simulink model "EncoderTrackingLoop"  (R2022a)
settings: Solver=ode4  StartTime=0.0  StopTime=inf  FixedStep=1/100  RelTol=1e-3
undefined symbols (not defined in the file): DiscIntNeverNeededParam, National_Instruments, PCI
libraries: sldrtlib x3, simulink x2
settings Model: Creator=UTFPR  LastModifiedBy=ederh
settings DebuggingCC: UnconnectedInputMsg=warning  UnconnectedOutputMsg=warning  UnconnectedLineMsg=warning
settings HardwareCC: ProdBitPerLong=64  ProdHWDeviceType=Intel->x86-64 (Linux 64)
settings RTWCC: Description=Simulink Desktop Real-Time  SystemTargetFile=sldrt.tlc  TemplateMakefile=sldrt.tmf  RTWCompilerOptimization=on  DLArmComputeVersion=19.05
settings CodeAppCC: MaxIdLength=95
settings SimulinkDesktopRealTimeCC: TargetLibSuffix=_sldrt.a  TargetPreCompLibLocation=C:\Program Files\MATLAB\R2022a\toolbox\sldrt\lib\win64

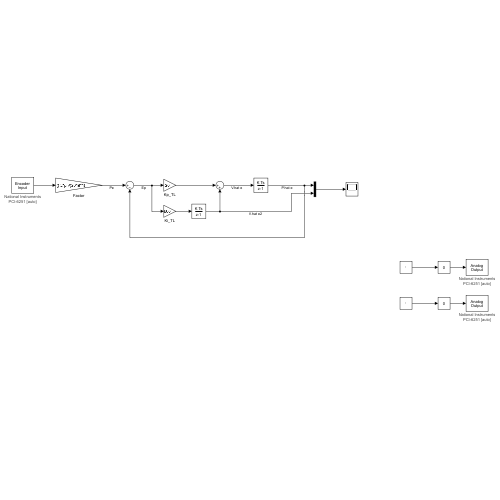
[thumbnail: Simulink's stored preview of the top-level diagram]
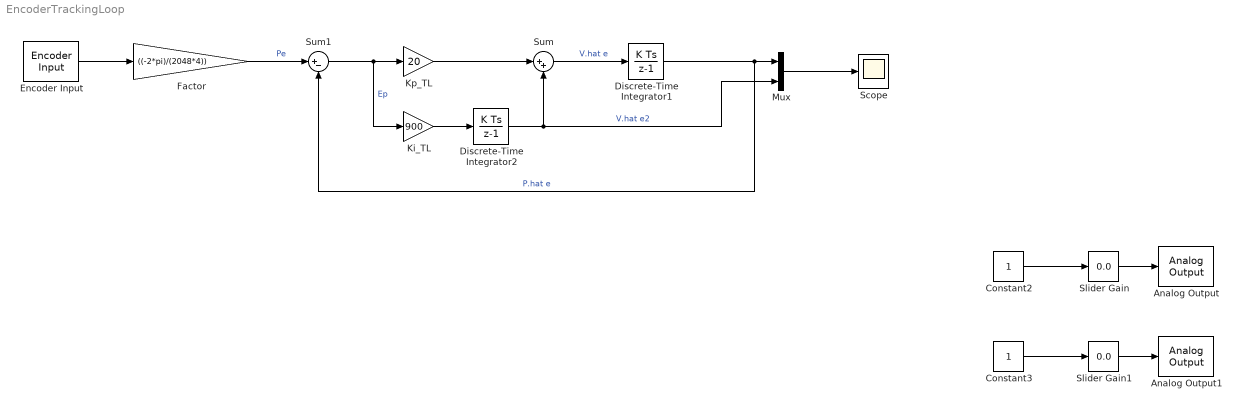
== system EncoderTrackingLoop ==
  Analog Output : sldrtlib/Analog Output  SampleTime=1/100  MaxMissedTicks=10  ShowMissedTicks=off  YieldWhenWaiting=off  DrvName=National_Instruments/PCI-6251  DrvAddress=4294967295  DrvOptions=[0 0 0 2 0]  Channels=1  RangeMode=1  VoltRange=1  InitialValue=0  FinalValue=0
      settings: AttributesFormatString=National Instruments\nPCI-6251 [auto]
  Analog Output1 : sldrtlib/Analog Output  SampleTime=1/100  MaxMissedTicks=10  ShowMissedTicks=off  YieldWhenWaiting=off  DrvName=National_Instruments/PCI-6251  DrvAddress=4294967295  DrvOptions=[0 0 0 2 0]  Channels=2  RangeMode=1  VoltRange=1  InitialValue=0  FinalValue=0
      settings: AttributesFormatString=National Instruments\nPCI-6251 [auto]
  Constant2 : Constant
  Constant3 : Constant
  Discrete-Time Integrator1 : DiscreteIntegrator  SampleTime=-1  ICPrevOutput=DiscIntNeverNeededParam  ICPrevScaledInput=DiscIntNeverNeededParam
  Discrete-Time Integrator2 : DiscreteIntegrator  SampleTime=-1  ICPrevOutput=DiscIntNeverNeededParam  ICPrevScaledInput=DiscIntNeverNeededParam
  Encoder Input : sldrtlib/Encoder Input  SampleTime=1/100  MaxMissedTicks=10  ShowMissedTicks=off  YieldWhenWaiting=off  DrvName=National_Instruments/PCI-6251  DrvAddress=4294967295  DrvOptions=[0 0 0 2 0]  Channels=1  QuadMode=3  IndexPulse=1  InputFilter=Inf  DataType=1
      settings: AttributesFormatString=National Instruments\nPCI-6251 [auto]
  Factor : Gain  Gain=((-2*pi)/(2048*4))
  Ki_TL : Gain  Gain=900
  Kp_TL : Gain  Gain=20
  Mux : Mux  Inputs=2
  Scope : Scope
  Slider Gain : simulink/Math Operations/Slider Gain  gain=0.0  low=0  high=10
  Slider Gain1 : simulink/Math Operations/Slider Gain  gain=0.0  low=0  high=10
  Sum : Sum  Inputs=|++
  Sum1 : Sum  Inputs=|+-
  wires:
  Slider Gain/1 -> Analog Output/1
  Constant2/1 -> Slider Gain/1
  Constant3/1 -> Slider Gain1/1
  Slider Gain1/1 -> Analog Output1/1
  Encoder Input/1 -> Factor/1
  Sum1/1 -> Kp_TL/1, Ki_TL/1  "Ep"
  Ki_TL/1 -> Discrete-Time Integrator2/1
  Discrete-Time Integrator1/1 -> Sum1/2, Mux/1  "P.hat e"
  Discrete-Time Integrator2/1 -> Sum/2, Mux/2  "V.hat e2"
  Kp_TL/1 -> Sum/1
  Factor/1 -> Sum1/1  "Pe"
  Sum/1 -> Discrete-Time Integrator1/1  "V.hat e"
  Mux/1 -> Scope/1
